simulink model "Band_shelf_12"  (R2024b)
settings: Solver=VariableStepAuto  StartTime=0.0  StopTime=10.0  RelTol=1e-3
libraries: dspsrcs4 x1
settings Model: Creator=woutlyen  LastModifiedBy=woutlyen

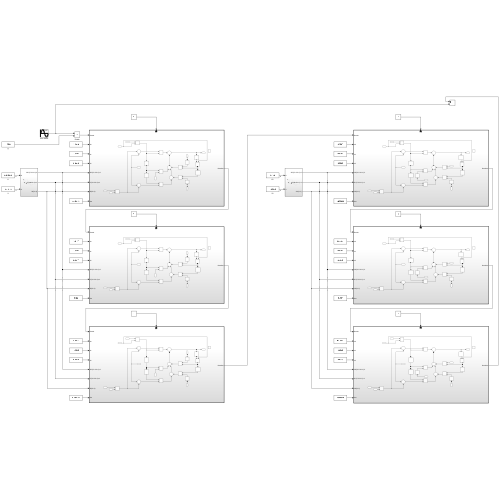
[thumbnail: Simulink's stored preview of the top-level diagram]
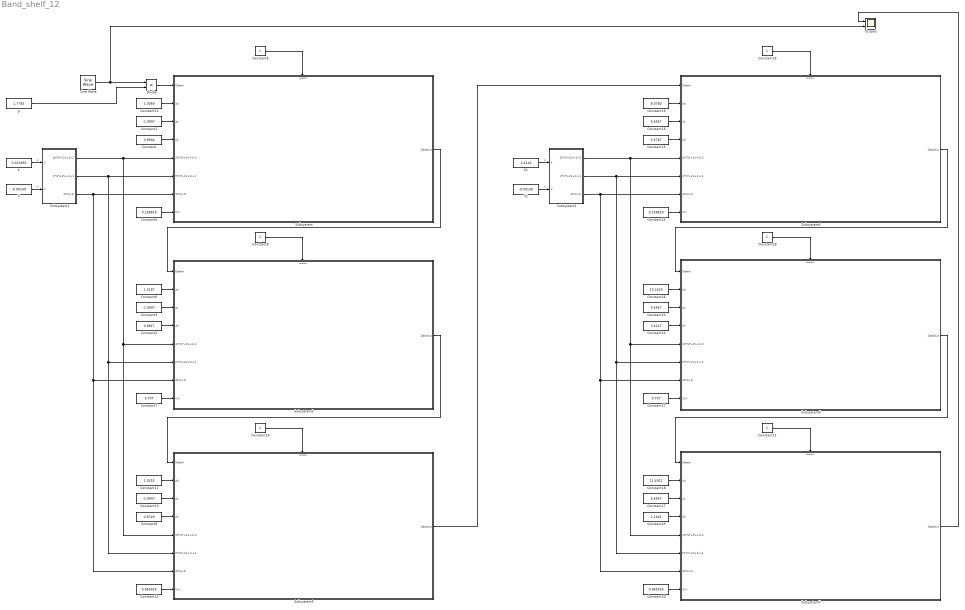
== system Band_shelf_12 ==
  Constant : Constant  Value=0.9934  OutDataTypeStr=fixdt(1,27,23)
  Constant1 : Constant  Value=-1.9997  OutDataTypeStr=fixdt(1,27,23)
  Constant10 : Constant  Value=-1.9997  OutDataTypeStr=fixdt(1,27,23)
  Constant11 : Constant  Value=1.0255  OutDataTypeStr=fixdt(1,27,23)
  Constant12 : Constant  Value=1.0069  OutDataTypeStr=fixdt(1,27,23)
  Constant13 : Constant  Value=0.965926  OutDataTypeStr=fixdt(1,27,23)
  Constant{5,8,14,21,25,28} (6 alike) : Constant  OutDataTypeStr=boolean
  Constant15 : Constant  Value=5.5787  OutDataTypeStr=fixdt(1,29,23)
  Constant16 : Constant  Value=9.6567  OutDataTypeStr=fixdt(1,29,23)
  Constant17 : Constant  Value=9.6567  OutDataTypeStr=fixdt(1,29,23)
  Constant18 : Constant  Value=11.4922  OutDataTypeStr=fixdt(1,29,23)
  Constant19 : Constant  Value=8.0780  OutDataTypeStr=fixdt(1,29,23)
  Constant2 : Constant  Value=0.9817  OutDataTypeStr=fixdt(1,27,23)
  Constant20 : Constant  Value=0.965926  OutDataTypeStr=fixdt(1,27,23)
  Constant22 : Constant  Value=3.4147  OutDataTypeStr=fixdt(1,29,23)
  Constant23 : Constant  Value=9.6567  OutDataTypeStr=fixdt(1,29,23)
  Constant24 : Constant  Value=0.258819  OutDataTypeStr=fixdt(1,27,23)
  Constant26 : Constant  Value=10.2420  OutDataTypeStr=fixdt(1,29,23)
  Constant27 : Constant  Value=0.707  OutDataTypeStr=fixdt(1,27,23)
  Constant29 : Constant  Value=2.1645  OutDataTypeStr=fixdt(1,29,23)
  Constant3 : Constant  Value=-1.9997  OutDataTypeStr=fixdt(1,27,23)
  Constant4 : Constant  Value=0.258819  OutDataTypeStr=fixdt(1,27,23)
  Constant6 : Constant  Value=1.0187  OutDataTypeStr=fixdt(1,27,23)
  Constant7 : Constant  Value=0.707  OutDataTypeStr=fixdt(1,27,23)
  Constant9 : Constant  Value=0.9749  OutDataTypeStr=fixdt(1,27,23)
  Divide : Product  Inputs=**  OutDataTypeStr=fixdt(1,27,23)
  K : Constant  Value=0.013091  OutDataTypeStr=fixdt(1,27,23)
  K1 : Constant  Value=2.4142  OutDataTypeStr=fixdt(1,27,23)
  Scope1 : Scope  NumInputPorts=2
  Sine Wave : dspsrcs4/Sine Wave  Amplitude=0.5012  Frequency=3000  Phase=0  SampleMode=Discrete  OutComplex=Real  CompMethod=Table lookup  TableSize=Speed  SampleTime=1/48000  SamplesPerFrame=1  ResetState=Restart at time zero  OutputFrames=off  dataType=Fixed-point  wordLen=24  udDataType=sfix(16)  fracBitsMode=User-defined  numFracBits=23  OutDataTypeStr=fixdt(1,24,23)  LastOutDataTypeStr=fixdt(1,24,23)
  Subsystem : Subsystem
  Subsystem1 : Subsystem
  Subsystem2 : Subsystem
  Subsystem3 : Subsystem
  Subsystem4 : Subsystem
  Subsystem5 : Subsystem
  Subsystem6 : Subsystem
  Subsystem7 : Subsystem
  V : Constant  Value=-0.09149  OutDataTypeStr=fixdt(1,27,23)
  V1 : Constant  Value=-0.09149  OutDataTypeStr=fixdt(1,27,23)
  g : Constant  Value=1.7783  OutDataTypeStr=fixdt(1,27,23)
  wires:
  Constant1/1 -> Subsystem/3(a1)
  Sine Wave/1 -> Divide/1, Scope1/2
  Constant5/1 -> Subsystem/Enable
  Constant12/1 -> Subsystem/2(a0)
  Subsystem1/2(K²(V²+2V+1)+1) -> Subsystem/6(K²(V²+2V+1)+1), Subsystem3/6(K²(V²+2V+1)+1), Subsystem2/6(K²(V²+2V+1)+1)
  Constant9/1 -> Subsystem3/4(a2)
  Subsystem2/1(DataOut) -> Subsystem3/1(DataIn)
  V/1 -> Subsystem1/2(V)  "V"
  K/1 -> Subsystem1/1(K)  "K"
  Constant8/1 -> Subsystem2/Enable
  Constant10/1 -> Subsystem3/3(a1)
  Constant13/1 -> Subsystem3/8(Cm)
  Constant11/1 -> Subsystem3/2(a0)
  Constant4/1 -> Subsystem/8(Cm)
  Constant3/1 -> Subsystem2/3(a1)
  Constant7/1 -> Subsystem2/8(Cm)
  Subsystem/1(DataOut) -> Subsystem2/1(DataIn)
  Constant6/1 -> Subsystem2/2(a0)
  Constant14/1 -> Subsystem3/Enable
  Constant2/1 -> Subsystem2/4(a2)
  Subsystem1/1(2K²(V²+2V+1)-2) -> Subsystem/5(2K²(V²+2V+1)-2), Subsystem3/5(2K²(V²+2V+1)-2), Subsystem2/5(2K²(V²+2V+1)-2)
  Subsystem1/3(2K(V+1)) -> Subsystem/7(2K(V+1)), Subsystem3/7(2K(V+1)), Subsystem2/7(2K(V+1))
  Constant/1 -> Subsystem/4(a2)
  Subsystem6/1(DataOut) -> Subsystem7/1(DataIn)
  Subsystem5/3(2K(V+1)) -> Subsystem4/7(2K(V+1)), Subsystem7/7(2K(V+1)), Subsystem6/7(2K(V+1))
  Subsystem7/1(DataOut) -> Scope1/1
  Constant19/1 -> Subsystem4/2(a0)
  Constant20/1 -> Subsystem7/8(Cm)
  Constant21/1 -> Subsystem7/Enable
  Constant24/1 -> Subsystem4/8(Cm)
  K1/1 -> Subsystem5/1(K)  "K"
  Constant15/1 -> Subsystem4/4(a2)
  Subsystem5/2(K²(V²+2V+1)+1) -> Subsystem4/6(K²(V²+2V+1)+1), Subsystem7/6(K²(V²+2V+1)+1), Subsystem6/6(K²(V²+2V+1)+1)
  Constant28/1 -> Subsystem6/Enable
  Constant27/1 -> Subsystem6/8(Cm)
  Constant17/1 -> Subsystem7/3(a1)
  V1/1 -> Subsystem5/2(V)  "V"
  Constant29/1 -> Subsystem7/4(a2)
  Constant23/1 -> Subsystem6/3(a1)
  Constant18/1 -> Subsystem7/2(a0)
  Constant22/1 -> Subsystem6/4(a2)
  Subsystem4/1(DataOut) -> Subsystem6/1(DataIn)
  Constant26/1 -> Subsystem6/2(a0)
  Subsystem5/1(2K²(V²+2V+1)-2) -> Subsystem4/5(2K²(V²+2V+1)-2), Subsystem7/5(2K²(V²+2V+1)-2), Subsystem6/5(2K²(V²+2V+1)-2)
  Constant25/1 -> Subsystem4/Enable
  Constant16/1 -> Subsystem4/3(a1)
  Subsystem3/1(DataOut) -> Subsystem4/1(DataIn)
  Divide/1 -> Subsystem/1(DataIn)
  g/1 -> Divide/2

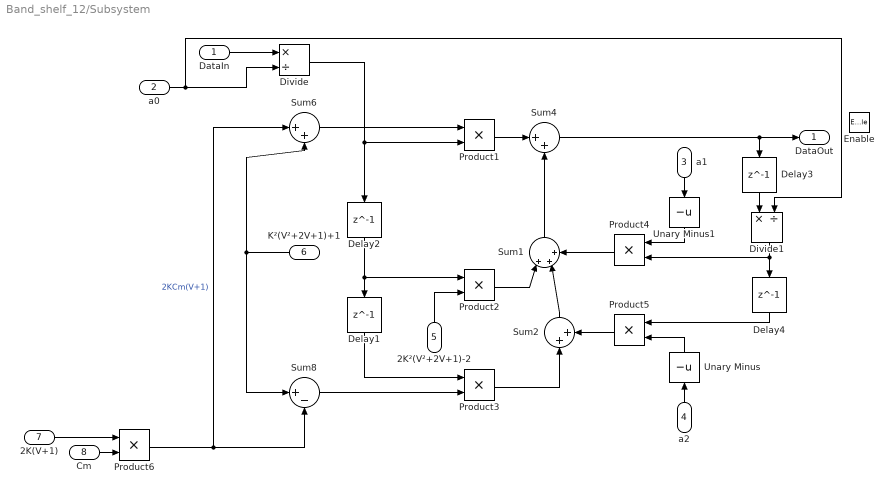
== system Band_shelf_12/Subsystem ==
  DataIn : Inport
  a0 : Inport  Port=2
  a1 : Inport  Port=3
  a2 : Inport  Port=4
  2K²(V²+2V+1)-2 : Inport  Port=5
  K²(V²+2V+1)+1 : Inport  Port=6
  2K(V+1) : Inport  Port=7
  Cm : Inport  Port=8
  Enable : EnablePort
  Delay{1..4} (4 alike) : Delay  DelayLength=1  InitialCondition=0
  Divide : Product  Inputs=*/  OutDataTypeStr=fixdt(1,27,23)
  Divide1 : Product  Inputs=*/  OutDataTypeStr=fixdt(1,27,23)
  Product{1..6} (6 alike) : Product  OutDataTypeStr=fixdt(1,27,23)
  Sum1 : Sum  Inputs=|+++
  Sum2 : Sum  Inputs=|++
  Sum4 : Sum  Inputs=|++
  Sum6 : Sum  Inputs=|++
  Sum8 : Sum  Inputs=|+-
  Unary Minus : UnaryMinus
  Unary Minus1 : UnaryMinus
  DataOut : Outport  VectorParamsAs1DForOutWhenUnconnected=off
  wires:
  Sum1/1 -> Sum4/2
  Product5/1 -> Sum2/2
  a1/1 -> Unary Minus1/1
  Unary Minus1/1 -> Product4/1
  Delay3/1 -> Divide1/1
  DataIn/1 -> Divide/1
  Product3/1 -> Sum2/1
  a0/1 -> Divide/2, Divide1/2
  K²(V²+2V+1)+1/1 -> Sum8/1, Sum6/2
  Unary Minus/1 -> Product5/2
  2K(V+1)/1 -> Product6/1
  Sum4/1 -> DataOut/1, Delay3/1
  Delay4/1 -> Product5/1
  Sum6/1 -> Product1/1
  2K²(V²+2V+1)-2/1 -> Product2/2
  Sum8/1 -> Product3/2
  Product6/1 -> Sum6/1, Sum8/2  "2KCm(V+1)"
  Divide1/1 -> Product4/2, Delay4/1
  Product2/1 -> Sum1/1
  Product4/1 -> Sum1/3
  Delay1/1 -> Product3/1
  Delay2/1 -> Product2/1, Delay1/1
  a2/1 -> Unary Minus/1
  Sum2/1 -> Sum1/2
  Divide/1 -> Product1/2, Delay2/1
  Cm/1 -> Product6/2
  Product1/1 -> Sum4/1

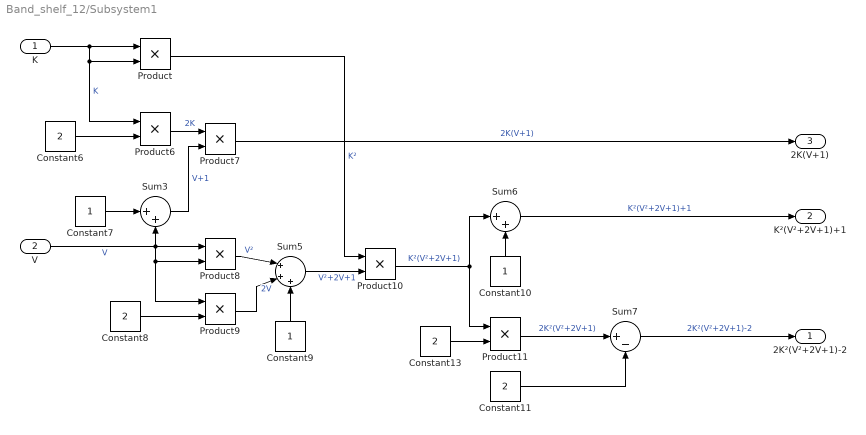
== system Band_shelf_12/Subsystem1 ==
  K : Inport
  V : Inport  Port=2
  Constant10 : Constant  SampleTime=-1
  Constant{6,8,11,13} (4 alike) : Constant  Value=2  SampleTime=-1
  Constant7 : Constant  SampleTime=-1
  Constant9 : Constant  SampleTime=-1
  Product{,6..11} (7 alike) : Product  OutDataTypeStr=fixdt(1,27,23)
  Sum3 : Sum  Inputs=|++
  Sum5 : Sum  Inputs=|+++
  Sum6 : Sum  Inputs=|++
  Sum7 : Sum  Inputs=|+-
  2K²(V²+2V+1)-2 : Outport
  K²(V²+2V+1)+1 : Outport  Port=2
  2K(V+1) : Outport  Port=3
  wires:
  Constant8/1 -> Product9/2
  Product11/1 -> Sum7/1  "2K²(V²+2V+1)"
  Constant7/1 -> Sum3/1
  Constant10/1 -> Sum6/2
  Sum3/1 -> Product7/2  "V+1"
  Constant9/1 -> Sum5/3
  Sum6/1 -> K²(V²+2V+1)+1/1  "K²(V²+2V+1)+1"
  Product10/1 -> Sum6/1, Product11/1  "K²(V²+2V+1)"
  Sum5/1 -> Product10/2  "V²+2V+1"
  Constant11/1 -> Sum7/2
  Product6/1 -> Product7/1  "2K"
  Product7/1 -> 2K(V+1)/1  "2K(V+1)"
  V/1 -> Product9/1, Product8/2, Product8/1, Sum3/2  "V"
  Sum7/1 -> 2K²(V²+2V+1)-2/1  "2K²(V²+2V+1)-2"
  K/1 -> Product6/1, Product/2, Product/1  "K"
  Constant6/1 -> Product6/2
  Product8/1 -> Sum5/1  "V²"
  Constant13/1 -> Product11/2
  Product9/1 -> Sum5/2  "2V"
  Product/1 -> Product10/1  "K²"

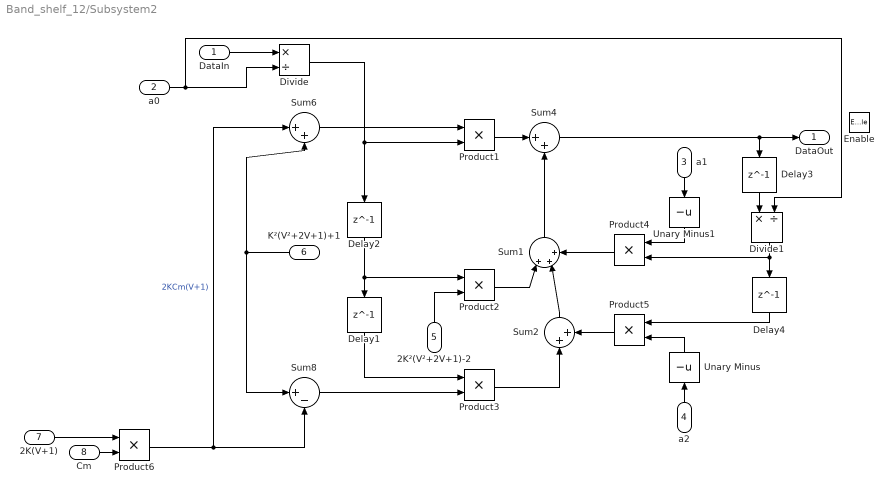
== system Band_shelf_12/Subsystem2 ==
  DataIn : Inport
  a0 : Inport  Port=2
  a1 : Inport  Port=3
  a2 : Inport  Port=4
  2K²(V²+2V+1)-2 : Inport  Port=5
  K²(V²+2V+1)+1 : Inport  Port=6
  2K(V+1) : Inport  Port=7
  Cm : Inport  Port=8
  Enable : EnablePort
  Delay{1..4} (4 alike) : Delay  DelayLength=1  InitialCondition=0
  Divide : Product  Inputs=*/  OutDataTypeStr=fixdt(1,27,23)
  Divide1 : Product  Inputs=*/  OutDataTypeStr=fixdt(1,27,23)
  Product{1..6} (6 alike) : Product  OutDataTypeStr=fixdt(1,27,23)
  Sum1 : Sum  Inputs=|+++
  Sum2 : Sum  Inputs=|++
  Sum4 : Sum  Inputs=|++
  Sum6 : Sum  Inputs=|++
  Sum8 : Sum  Inputs=|+-
  Unary Minus : UnaryMinus
  Unary Minus1 : UnaryMinus
  DataOut : Outport  VectorParamsAs1DForOutWhenUnconnected=off
  wires:
  Sum6/1 -> Product1/1
  Product6/1 -> Sum6/1, Sum8/2  "2KCm(V+1)"
  Product1/1 -> Sum4/1
  a0/1 -> Divide/2, Divide1/2
  Sum8/1 -> Product3/2
  Sum4/1 -> DataOut/1, Delay3/1
  Divide/1 -> Product1/2, Delay2/1
  Cm/1 -> Product6/2
  Unary Minus/1 -> Product5/2
  Delay4/1 -> Product5/1
  Unary Minus1/1 -> Product4/1
  Divide1/1 -> Product4/2, Delay4/1
  2K(V+1)/1 -> Product6/1
  Product3/1 -> Sum2/1
  Product2/1 -> Sum1/1
  Delay1/1 -> Product3/1
  Product4/1 -> Sum1/3
  Sum1/1 -> Sum4/2
  a1/1 -> Unary Minus1/1
  K²(V²+2V+1)+1/1 -> Sum8/1, Sum6/2
  Sum2/1 -> Sum1/2
  a2/1 -> Unary Minus/1
  Product5/1 -> Sum2/2
  2K²(V²+2V+1)-2/1 -> Product2/2
  Delay3/1 -> Divide1/1
  DataIn/1 -> Divide/1
  Delay2/1 -> Product2/1, Delay1/1

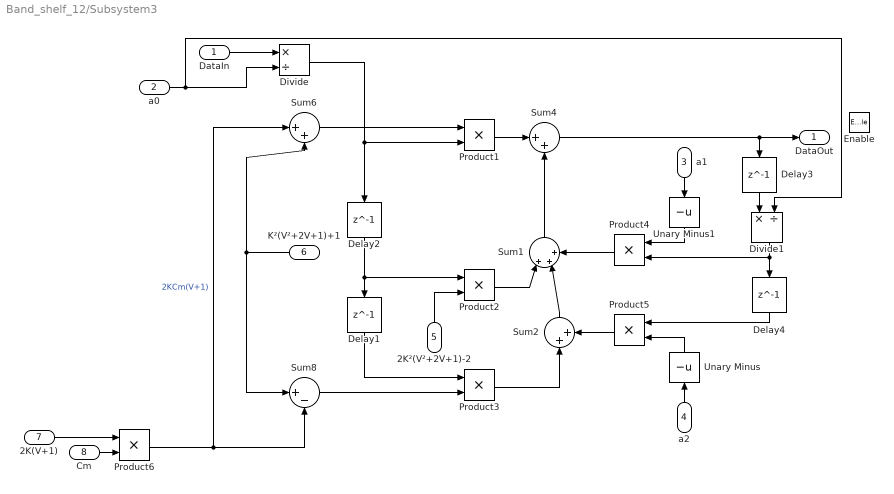
== system Band_shelf_12/Subsystem3 ==
  DataIn : Inport
  a0 : Inport  Port=2
  a1 : Inport  Port=3
  a2 : Inport  Port=4
  2K²(V²+2V+1)-2 : Inport  Port=5
  K²(V²+2V+1)+1 : Inport  Port=6
  2K(V+1) : Inport  Port=7
  Cm : Inport  Port=8
  Enable : EnablePort
  Delay{1..4} (4 alike) : Delay  DelayLength=1  InitialCondition=0
  Divide : Product  Inputs=*/  OutDataTypeStr=fixdt(1,27,23)
  Divide1 : Product  Inputs=*/  OutDataTypeStr=fixdt(1,27,23)
  Product{1..6} (6 alike) : Product  OutDataTypeStr=fixdt(1,27,23)
  Sum1 : Sum  Inputs=|+++
  Sum2 : Sum  Inputs=|++
  Sum4 : Sum  Inputs=|++
  Sum6 : Sum  Inputs=|++
  Sum8 : Sum  Inputs=|+-
  Unary Minus : UnaryMinus
  Unary Minus1 : UnaryMinus
  DataOut : Outport  VectorParamsAs1DForOutWhenUnconnected=off
  wires:
  Sum6/1 -> Product1/1
  Product6/1 -> Sum6/1, Sum8/2  "2KCm(V+1)"
  Product1/1 -> Sum4/1
  a0/1 -> Divide/2, Divide1/2
  Sum8/1 -> Product3/2
  Sum4/1 -> DataOut/1, Delay3/1
  Divide/1 -> Product1/2, Delay2/1
  Cm/1 -> Product6/2
  Unary Minus/1 -> Product5/2
  Delay4/1 -> Product5/1
  Unary Minus1/1 -> Product4/1
  Divide1/1 -> Product4/2, Delay4/1
  2K(V+1)/1 -> Product6/1
  Product3/1 -> Sum2/1
  Product2/1 -> Sum1/1
  Delay1/1 -> Product3/1
  Product4/1 -> Sum1/3
  Sum1/1 -> Sum4/2
  a1/1 -> Unary Minus1/1
  K²(V²+2V+1)+1/1 -> Sum8/1, Sum6/2
  Sum2/1 -> Sum1/2
  a2/1 -> Unary Minus/1
  Product5/1 -> Sum2/2
  2K²(V²+2V+1)-2/1 -> Product2/2
  Delay3/1 -> Divide1/1
  DataIn/1 -> Divide/1
  Delay2/1 -> Product2/1, Delay1/1

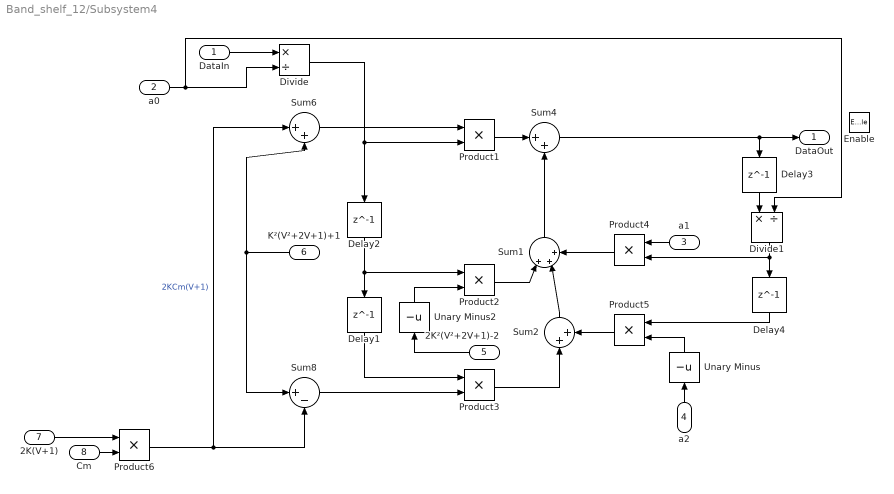
== system Band_shelf_12/Subsystem4 ==
  DataIn : Inport
  a0 : Inport  Port=2
  a1 : Inport  Port=3
  a2 : Inport  Port=4
  2K²(V²+2V+1)-2 : Inport  Port=5
  K²(V²+2V+1)+1 : Inport  Port=6
  2K(V+1) : Inport  Port=7
  Cm : Inport  Port=8
  Enable : EnablePort
  Delay{1..4} (4 alike) : Delay  DelayLength=1  InitialCondition=0
  Divide : Product  Inputs=*/  OutDataTypeStr=fixdt(1,29,23)
  Divide1 : Product  Inputs=*/  OutDataTypeStr=fixdt(1,27,23)
  Product{1..5} (5 alike) : Product  OutDataTypeStr=fixdt(1,27,23)
  Product6 : Product  OutDataTypeStr=fixdt(1,29,23)
  Sum1 : Sum  Inputs=|+++
  Sum2 : Sum  Inputs=|++
  Sum4 : Sum  Inputs=|++
  Sum6 : Sum  Inputs=|++
  Sum8 : Sum  Inputs=|+-
  Unary Minus : UnaryMinus
  Unary Minus2 : UnaryMinus
  DataOut : Outport  VectorParamsAs1DForOutWhenUnconnected=off
  wires:
  Sum1/1 -> Sum4/2
  Product5/1 -> Sum2/2
  a1/1 -> Product4/1
  Delay3/1 -> Divide1/1
  DataIn/1 -> Divide/1
  Product3/1 -> Sum2/1
  a0/1 -> Divide/2, Divide1/2
  K²(V²+2V+1)+1/1 -> Sum8/1, Sum6/2
  Unary Minus/1 -> Product5/2
  2K(V+1)/1 -> Product6/1
  Sum4/1 -> DataOut/1, Delay3/1
  Delay4/1 -> Product5/1
  Sum6/1 -> Product1/1
  2K²(V²+2V+1)-2/1 -> Unary Minus2/1
  Sum8/1 -> Product3/2
  Product6/1 -> Sum6/1, Sum8/2  "2KCm(V+1)"
  Divide1/1 -> Product4/2, Delay4/1
  Product2/1 -> Sum1/1
  Product4/1 -> Sum1/3
  Delay1/1 -> Product3/1
  Delay2/1 -> Delay1/1, Product2/1
  a2/1 -> Unary Minus/1
  Sum2/1 -> Sum1/2
  Divide/1 -> Product1/2, Delay2/1
  Cm/1 -> Product6/2
  Product1/1 -> Sum4/1
  Unary Minus2/1 -> Product2/2

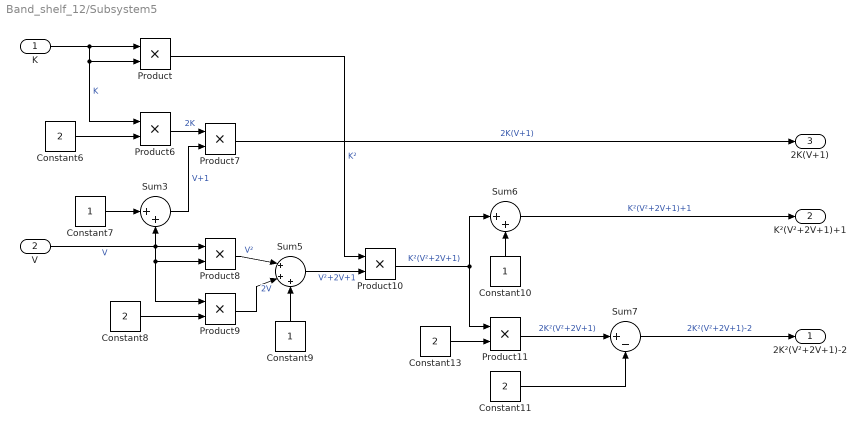
== system Band_shelf_12/Subsystem5 ==
  K : Inport
  V : Inport  Port=2
  Constant10 : Constant  SampleTime=-1
  Constant{6,8,11,13} (4 alike) : Constant  Value=2  SampleTime=-1
  Constant7 : Constant  SampleTime=-1
  Constant9 : Constant  SampleTime=-1
  Product{,6..11} (7 alike) : Product  OutDataTypeStr=fixdt(1,29,23)
  Sum3 : Sum  Inputs=|++
  Sum5 : Sum  Inputs=|+++
  Sum6 : Sum  Inputs=|++
  Sum7 : Sum  Inputs=|+-
  2K²(V²+2V+1)-2 : Outport
  K²(V²+2V+1)+1 : Outport  Port=2
  2K(V+1) : Outport  Port=3
  wires:
  Constant8/1 -> Product9/2
  Product11/1 -> Sum7/1  "2K²(V²+2V+1)"
  Constant7/1 -> Sum3/1
  Constant10/1 -> Sum6/2
  Sum3/1 -> Product7/2  "V+1"
  Constant9/1 -> Sum5/3
  Sum6/1 -> K²(V²+2V+1)+1/1  "K²(V²+2V+1)+1"
  Product10/1 -> Sum6/1, Product11/1  "K²(V²+2V+1)"
  Sum5/1 -> Product10/2  "V²+2V+1"
  Constant11/1 -> Sum7/2
  Product6/1 -> Product7/1  "2K"
  Product7/1 -> 2K(V+1)/1  "2K(V+1)"
  V/1 -> Product9/1, Product8/2, Product8/1, Sum3/2  "V"
  Sum7/1 -> 2K²(V²+2V+1)-2/1  "2K²(V²+2V+1)-2"
  K/1 -> Product6/1, Product/2, Product/1  "K"
  Constant6/1 -> Product6/2
  Product8/1 -> Sum5/1  "V²"
  Constant13/1 -> Product11/2
  Product9/1 -> Sum5/2  "2V"
  Product/1 -> Product10/1  "K²"

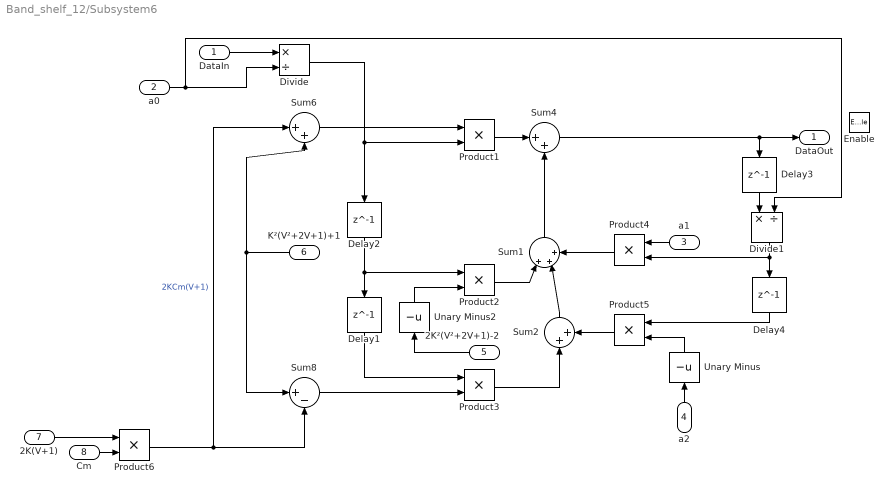
== system Band_shelf_12/Subsystem6 ==
  DataIn : Inport
  a0 : Inport  Port=2
  a1 : Inport  Port=3
  a2 : Inport  Port=4
  2K²(V²+2V+1)-2 : Inport  Port=5
  K²(V²+2V+1)+1 : Inport  Port=6
  2K(V+1) : Inport  Port=7
  Cm : Inport  Port=8
  Enable : EnablePort
  Delay{1..4} (4 alike) : Delay  DelayLength=1  InitialCondition=0
  Divide : Product  Inputs=*/  OutDataTypeStr=fixdt(1,29,23)
  Divide1 : Product  Inputs=*/  OutDataTypeStr=fixdt(1,27,23)
  Product{1..5} (5 alike) : Product  OutDataTypeStr=fixdt(1,27,23)
  Product6 : Product  OutDataTypeStr=fixdt(1,29,23)
  Sum1 : Sum  Inputs=|+++
  Sum2 : Sum  Inputs=|++
  Sum4 : Sum  Inputs=|++
  Sum6 : Sum  Inputs=|++
  Sum8 : Sum  Inputs=|+-
  Unary Minus : UnaryMinus
  Unary Minus2 : UnaryMinus
  DataOut : Outport  VectorParamsAs1DForOutWhenUnconnected=off
  wires:
  Sum8/1 -> Product3/2
  a1/1 -> Product4/1
  Sum4/1 -> DataOut/1, Delay3/1
  Delay2/1 -> Delay1/1, Product2/1
  Sum6/1 -> Product1/1
  Sum2/1 -> Sum1/2
  Unary Minus2/1 -> Product2/2
  Unary Minus/1 -> Product5/2
  Delay4/1 -> Product5/1
  2K(V+1)/1 -> Product6/1
  DataIn/1 -> Divide/1
  Product6/1 -> Sum6/1, Sum8/2  "2KCm(V+1)"
  Product2/1 -> Sum1/1
  Sum1/1 -> Sum4/2
  2K²(V²+2V+1)-2/1 -> Unary Minus2/1
  Delay3/1 -> Divide1/1
  Cm/1 -> Product6/2
  Product1/1 -> Sum4/1
  Divide1/1 -> Product4/2, Delay4/1
  Product3/1 -> Sum2/1
  Divide/1 -> Product1/2, Delay2/1
  Delay1/1 -> Product3/1
  Product4/1 -> Sum1/3
  Product5/1 -> Sum2/2
  a2/1 -> Unary Minus/1
  a0/1 -> Divide/2, Divide1/2
  K²(V²+2V+1)+1/1 -> Sum8/1, Sum6/2

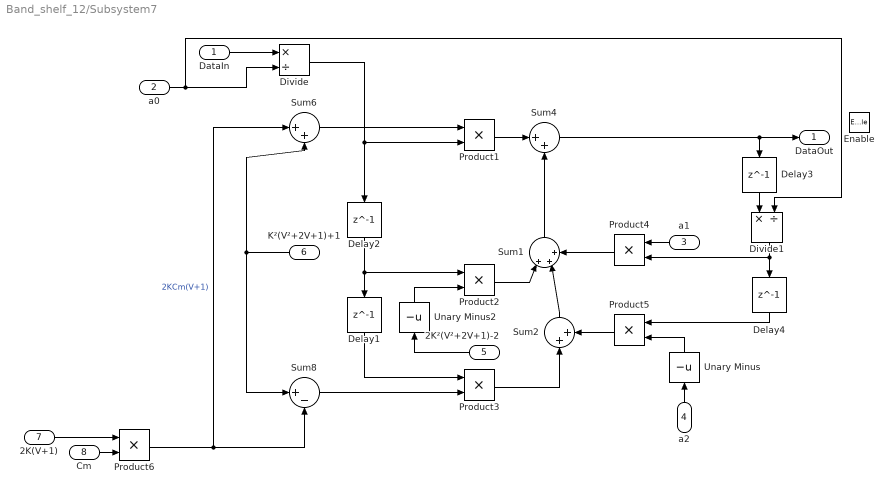
== system Band_shelf_12/Subsystem7 ==
  DataIn : Inport
  a0 : Inport  Port=2
  a1 : Inport  Port=3
  a2 : Inport  Port=4
  2K²(V²+2V+1)-2 : Inport  Port=5
  K²(V²+2V+1)+1 : Inport  Port=6
  2K(V+1) : Inport  Port=7
  Cm : Inport  Port=8
  Enable : EnablePort
  Delay{1..4} (4 alike) : Delay  DelayLength=1  InitialCondition=0
  Divide : Product  Inputs=*/  OutDataTypeStr=fixdt(1,29,23)
  Divide1 : Product  Inputs=*/  OutDataTypeStr=fixdt(1,29,23)
  Product{1..6} (6 alike) : Product  OutDataTypeStr=fixdt(1,29,23)
  Sum1 : Sum  Inputs=|+++
  Sum2 : Sum  Inputs=|++
  Sum4 : Sum  Inputs=|++
  Sum6 : Sum  Inputs=|++
  Sum8 : Sum  Inputs=|+-
  Unary Minus : UnaryMinus
  Unary Minus2 : UnaryMinus
  DataOut : Outport  VectorParamsAs1DForOutWhenUnconnected=off
  wires:
  Sum8/1 -> Product3/2
  a1/1 -> Product4/1
  Sum4/1 -> DataOut/1, Delay3/1
  Delay2/1 -> Delay1/1, Product2/1
  Sum6/1 -> Product1/1
  Sum2/1 -> Sum1/2
  Unary Minus2/1 -> Product2/2
  Unary Minus/1 -> Product5/2
  Delay4/1 -> Product5/1
  2K(V+1)/1 -> Product6/1
  DataIn/1 -> Divide/1
  Product6/1 -> Sum6/1, Sum8/2  "2KCm(V+1)"
  Product2/1 -> Sum1/1
  Sum1/1 -> Sum4/2
  2K²(V²+2V+1)-2/1 -> Unary Minus2/1
  Delay3/1 -> Divide1/1
  Cm/1 -> Product6/2
  Product1/1 -> Sum4/1
  Divide1/1 -> Product4/2, Delay4/1
  Product3/1 -> Sum2/1
  Divide/1 -> Product1/2, Delay2/1
  Delay1/1 -> Product3/1
  Product4/1 -> Sum1/3
  Product5/1 -> Sum2/2
  a2/1 -> Unary Minus/1
  a0/1 -> Divide/2, Divide1/2
  K²(V²+2V+1)+1/1 -> Sum8/1, Sum6/2
